simulink model "Primerpunto_b"  (R2017b)
settings: Solver=VariableStepAuto  StartTime=0.0  StopTime=5500  RelTol=1e-3
values from neighbouring files (symbols this model uses):
  a1 = 0.5    [PrimerPunto_b.m]
  a2 = 3.5    [PrimerPunto_b.m]
  m1 = 5    [PrimerPunto_b.m]
  m2 = 6    [PrimerPunto_b.m]
  r1 = 4    [PrimerPunto_b.m]
  r2 = 4    [PrimerPunto_b.m]
  s0 = 0.3    [PrimerPunto_b.m]
settings Model: Creator=HP  LastModifiedBy=franj
settings CodeAppCC: StateflowObjectComments=on

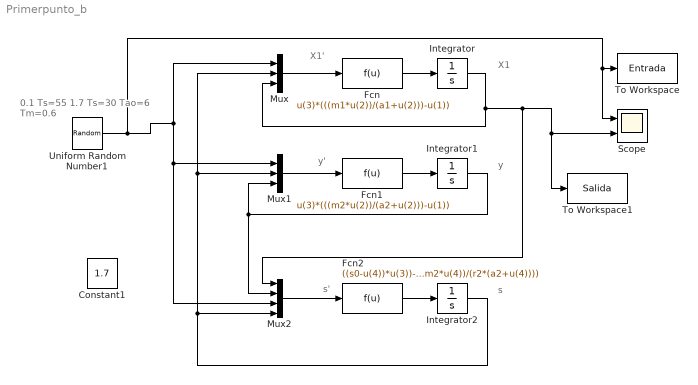
== system Primerpunto_b ==
  note: 0.1 Ts=55
      | 1.7 Ts=30
      | Tao=6
      | Tm=0.6
  note: s
  note: s'
  note: y
  note: X1'
  note: X1
  note: y'
  Constant1 : Constant  Value=1.7
  Fcn : Fcn  Expr=u(3)*(((m1*u(2))/(a1+u(2)))-u(1))
  Fcn1 : Fcn  Expr=u(3)*(((m2*u(2))/(a2+u(2)))-u(1))
  Fcn2 : Fcn  Expr=((s0-u(4))*u(3))-((u(1)*m1*u(4))/(r1*(a1+u(4))))-((u(2)*m2*u(4))/(r2*(a2+u(4))))
  Integrator : Integrator  InitialCondition=0.1
  Integrator1 : Integrator
  Integrator2 : Integrator
  Mux : Mux  Inputs=3
  Mux1 : Mux  Inputs=3
  Mux2 : Mux
  Scope : Scope  NumInputPorts=2
  To Workspace : ToWorkspace  VariableName=Entrada  SampleTime=0.9
  To Workspace1 : ToWorkspace  VariableName=Salida  SampleTime=0.9
  Uniform Random Number1 : UniformRandomNumber  Minimum=0.1  Maximum=1.7  SampleTime=55
  wires:
  Mux/1 -> Fcn/1
  Uniform Random Number1/1 -> Scope/1, To Workspace/1, Mux/1, Mux2/3, Mux1/1
  Fcn1/1 -> Integrator1/1
  Fcn2/1 -> Integrator2/1
  Fcn/1 -> Integrator/1
  Integrator/1 -> Scope/2, To Workspace1/1, Mux2/1, Mux/3
  Integrator2/1 -> Mux2/4, Mux1/2, Mux/2
  Integrator1/1 -> Mux2/2, Mux1/3
  Mux1/1 -> Fcn1/1
  Mux2/1 -> Fcn2/1
